simulink model "dqn_C_PQ_HVsMC"  (R2024a)
settings: Solver=FixedStepDiscrete  StartTime=0.0  StopTime=10  FixedStep=Ts_Power  RelTol=1e-3
PreLoadFcn:
  | % HVDCMMCInterconnectionParam
StartFcn:
  | tic
StopFcn:
  | toc
values from neighbouring files (symbols this model uses):
  C_PM = 1.758e-3    (= 0.001758)    [dqnMMCsingle.m]
  Fnom = 50    [dqnMMCsingle.m]
  Ki_Ireg = 6    [dqnMMCsingle.m]
  Ki_Qreg = 1.0    (= 1)    [dqnMMCsingle.m]
  Kp_Ireg = 0.6    [dqnMMCsingle.m]
  Kp_Qreg = 0.5/3    (= 0.166666666667)    [dqnMMCsingle.m]
  Larm = Larm_pu*(Zb_ac/(2*pi*Fnom))    [dqnMMCsingle.m]
  Larm_pu = 0.15    [dqnMMCsingle.m]
  Lff = Larm_pu/2    (= 0.075)    [dqnMMCsingle.m]
  Limits_Ireg = [ 2.0  -2.0]    [dqnMMCsingle.m]
  Limits_Qreg = [ 0.25, -0.25 ]    [dqnMMCsingle.m]
  Limits_VDCreg = [ 2.0  -2.0]    [dqnMMCsingle.m]
  Lxfo = 0.12    [dqnMMCsingle.m]
  N = 1    [dqnMMCsingle.m]
  Nb_PM = 36    [dqnMMCsingle.m]
  Pnom = 1000e6    (= 1000000000)    [dqnMMCsingle.m]
  R_startup = 400    [dqnMMCsingle.m]
  Rarm = Rarm_pu*Zb_ac    [dqnMMCsingle.m]
  Rff = Rarm_pu/2    (= 0.00075)    [dqnMMCsingle.m]
  Rxfo = 0.003    [dqnMMCsingle.m]
  Slope_Qref = 0.5    [dqnMMCsingle.m]
  Slope_Vdc_ref = Vnom_dc/5    (= 128000)    [dqnMMCsingle.m]
  Tfault = 9999    [dqnMMCsingle.m]
  Ts = Ts_Control    (= 4e-05)    [dqnMMCsingle.m]
  Ts_Control = 40e-6    (= 4e-05)    [dqnMMCsingle.m]
  Ts_dqn = 2e-5    (= 2e-05)    [dqnMMCsingle.m]
  Ts_Power = 20e-6    (= 2e-05)    [dqnMMCsingle.m]
  Vnom_dc = 640e3    (= 640000)    [dqnMMCsingle.m]
  Vnom_prim = 400e3    (= 400000)    [dqnMMCsingle.m]
  Vnom_sec = 333e3    (= 333000)    [dqnMMCsingle.m]
undefined symbols (not defined in the file or in its folder): DiscIntNeverNeededParam, Discrete, DQN_Lib, gcbh, HRM, Int_DQNc_Mat, Mult_DQNc_Mat, Pcc, S, sps, sps_rtmsupport, spsMeanValueVariableFrequencyModel, spsPLL3phModel, SY3, Ws
libraries: simulink x18, spsControlledVoltageSourceLib x15, spsVoltageMeasurementLib x9, powerlib_extras x6, spsSecondOrderFilterLib x6, spsCurrentMeasurementLib x6, spsIdealSwitchLib x6, spsMeanLib x4, spsdq0toabcLib x4, spsMeanVariableFrequencyLib x4, spsabctodq0Lib x4, spsThreePhaseSeriesRLCBranchLib x4
(part 4 of 6)

== system dqn_C_PQ_HVsMC/Control _DQn/PLL, Measurements and Transformation1/PLL (3ph)/Model/Variable Frequency Mean value/Model/Correction subsystem ==
  N : Inport
  F : Inport  Port=2
  In : Inport  Port=3
  Gain1 : Gain  Gain=0.5  SaturateOnIntegerOverflow=on  OutDataTypeStr=Inherit: Same as input  ParamDataTypeStr=Inherit: Same as input
  Product2 : Product  Inputs=*/  InputSameDT=on  SaturateOnIntegerOverflow=on  OutDataTypeStr=Inherit: Same as first input
  Product4 : Product  Inputs=**  InputSameDT=on  SaturateOnIntegerOverflow=on  OutDataTypeStr=Inherit: Same as first input
  Product5 : Product  Inputs=**  InputSameDT=on  SaturateOnIntegerOverflow=on  OutDataTypeStr=Inherit: Same as first input
  Sum1 : Sum  Inputs=+-  InputSameDT=on  SaturateOnIntegerOverflow=on  OutDataTypeStr=Inherit: Same as first input
  Sum4 : Sum  InputSameDT=on  SaturateOnIntegerOverflow=on  OutDataTypeStr=Inherit: Same as first input
  Sum5 : Sum  Inputs=+-  InputSameDT=on  SaturateOnIntegerOverflow=on  OutDataTypeStr=Inherit: Same as first input
  Unit Delay : UnitDelay  SampleTime=Ts  HasFrameUpgradeWarning=on
  Out : Outport
  wires:
  Product4/1 -> Out/1
  Sum4/1 -> Product4/2
  Gain1/1 -> Sum4/1
  Product5/1 -> Gain1/1
  Sum1/1 -> Product5/2
  In/1 -> Sum4/2, Unit Delay/1, Sum1/1
  Product2/1 -> Product4/1
  Sum5/1 -> Product5/1, Product2/1
  F/1 -> Sum5/2
  N/1 -> Product2/2, Sum5/1
  Unit Delay/1 -> Sum1/2

== system dqn_C_PQ_HVsMC/Control _DQn/PLL, Measurements and Transformation1/PLL (3ph)2/Model/Variable Frequency Mean value/Model/Correction subsystem ==
  N : Inport
  F : Inport  Port=2
  In : Inport  Port=3
  Gain1 : Gain  Gain=0.5  SaturateOnIntegerOverflow=on  OutDataTypeStr=Inherit: Same as input  ParamDataTypeStr=Inherit: Same as input
  Product2 : Product  Inputs=*/  InputSameDT=on  SaturateOnIntegerOverflow=on  OutDataTypeStr=Inherit: Same as first input
  Product4 : Product  Inputs=**  InputSameDT=on  SaturateOnIntegerOverflow=on  OutDataTypeStr=Inherit: Same as first input
  Product5 : Product  Inputs=**  InputSameDT=on  SaturateOnIntegerOverflow=on  OutDataTypeStr=Inherit: Same as first input
  Sum1 : Sum  Inputs=+-  InputSameDT=on  SaturateOnIntegerOverflow=on  OutDataTypeStr=Inherit: Same as first input
  Sum4 : Sum  InputSameDT=on  SaturateOnIntegerOverflow=on  OutDataTypeStr=Inherit: Same as first input
  Sum5 : Sum  Inputs=+-  InputSameDT=on  SaturateOnIntegerOverflow=on  OutDataTypeStr=Inherit: Same as first input
  Unit Delay : UnitDelay  SampleTime=Ts  HasFrameUpgradeWarning=on
  Out : Outport
  wires:
  Product4/1 -> Out/1
  Sum4/1 -> Product4/2
  Gain1/1 -> Sum4/1
  Product5/1 -> Gain1/1
  Sum1/1 -> Product5/2
  In/1 -> Sum4/2, Unit Delay/1, Sum1/1
  Product2/1 -> Product4/1
  Sum5/1 -> Product5/1, Product2/1
  F/1 -> Sum5/2
  N/1 -> Product2/2, Sum5/1
  Unit Delay/1 -> Sum1/2

== matlab function dqn_C_PQ_HVsMC/DQsym/Subsystem/DQn->ABC11 ==
  settings: updateMethod=DISCRETE
  data: Xdcpnz_c input; tho input; Xabc output; N parameter
%function abc = Mult(Z0,Zdp,Zqp,Zdn,Zqn,Zdz,Zqz,th, N)
function Xabc = dqn2abc(Xdcpnz_c,tho,N)

    persistent Sas;
    persistent Ssa;

    if(isempty(Sas)) 
        a = -0.5+0.866i;
        a2 = -0.5-0.866i;
        Sas = [1,a,a2;1,a2,a;1,1,1]/3;
        Ssa = eye(3)/(Sas);
    end

    Xabc = zeros(3,1);

    for i = 1 : N+1
    
    
        if(i>1)
            h = i-1;
    
            th = h*tho;
        
            mag_p = abs(Xdcpnz_c(1,i));
            ang_p = angle(Xdcpnz_c(1,i));
            mag_n = abs(Xdcpnz_c(2,i));
            ang_n = angle(Xdcpnz_c(2,i));
            mag_z = abs(Xdcpnz_c(3,i));
            ang_z = angle(Xdcpnz_c(3,i));
            
            abc3p = mag_p*[sin(th+ang_p) ; sin(th+ang_p-2*pi/3) ; sin(th+ang_p+2*pi/3) ];
            abc3n = mag_n*[sin(th+ang_n) ; sin(th+ang_n+2*pi/3) ; sin(th+ang_n-2*pi/3) ];
            abc3z = mag_z*[sin(th+ang_z) ; sin(th+ang_z)        ; sin(th+ang_z)  ];
        
            Xabc = Xabc + abc3p+abc3n+abc3z;
        else
            Xabc = Xabc + real(Ssa*(Xdcpnz_c(:,1)));
        
        end
    
        
    end

end

== matlab function dqn_C_PQ_HVsMC/DQsym/Subsystem/DQn->ABC12 ==
  settings: updateMethod=DISCRETE
  data: Xdcpnz_c input; tho input; Xabc output; N parameter
%function abc = Mult(Z0,Zdp,Zqp,Zdn,Zqn,Zdz,Zqz,th, N)
function Xabc = dqn2abc(Xdcpnz_c,tho,N)

    persistent Sas;
    persistent Ssa;

    if(isempty(Sas)) 
        a = -0.5+0.866i;
        a2 = -0.5-0.866i;
        Sas = [1,a,a2;1,a2,a;1,1,1]/3;
        Ssa = eye(3)/(Sas);
    end

    Xabc = zeros(3,1);

    for i = 1 : N+1
    
    
        if(i>1)
            h = i-1;
    
            th = h*tho;
        
            mag_p = abs(Xdcpnz_c(1,i));
            ang_p = angle(Xdcpnz_c(1,i));
            mag_n = abs(Xdcpnz_c(2,i));
            ang_n = angle(Xdcpnz_c(2,i));
            mag_z = abs(Xdcpnz_c(3,i));
            ang_z = angle(Xdcpnz_c(3,i));
            
            abc3p = mag_p*[sin(th+ang_p) ; sin(th+ang_p-2*pi/3) ; sin(th+ang_p+2*pi/3) ];
            abc3n = mag_n*[sin(th+ang_n) ; sin(th+ang_n+2*pi/3) ; sin(th+ang_n-2*pi/3) ];
            abc3z = mag_z*[sin(th+ang_z) ; sin(th+ang_z)        ; sin(th+ang_z)  ];
        
            Xabc = Xabc + abc3p+abc3n+abc3z;
        else
            Xabc = Xabc + real(Ssa*(Xdcpnz_c(:,1)));
        
        end
    
        
    end

end

== matlab function dqn_C_PQ_HVsMC/DQsym/Subsystem/DQn->ABC13 ==
  settings: updateMethod=DISCRETE
  data: Xdcpnz_c input; tho input; Xabc output; N parameter
%function abc = Mult(Z0,Zdp,Zqp,Zdn,Zqn,Zdz,Zqz,th, N)
function Xabc = dqn2abc(Xdcpnz_c,tho,N)

    persistent Sas;
    persistent Ssa;

    if(isempty(Sas)) 
        a = -0.5+0.866i;
        a2 = -0.5-0.866i;
        Sas = [1,a,a2;1,a2,a;1,1,1]/3;
        Ssa = eye(3)/(Sas);
    end

    Xabc = zeros(3,1);

    for i = 1 : N+1
    
    
        if(i>1)
            h = i-1;
    
            th = h*tho;
        
            mag_p = abs(Xdcpnz_c(1,i));
            ang_p = angle(Xdcpnz_c(1,i));
            mag_n = abs(Xdcpnz_c(2,i));
            ang_n = angle(Xdcpnz_c(2,i));
            mag_z = abs(Xdcpnz_c(3,i));
            ang_z = angle(Xdcpnz_c(3,i));
            
            abc3p = mag_p*[sin(th+ang_p) ; sin(th+ang_p-2*pi/3) ; sin(th+ang_p+2*pi/3) ];
            abc3n = mag_n*[sin(th+ang_n) ; sin(th+ang_n+2*pi/3) ; sin(th+ang_n-2*pi/3) ];
            abc3z = mag_z*[sin(th+ang_z) ; sin(th+ang_z)        ; sin(th+ang_z)  ];
        
            Xabc = Xabc + abc3p+abc3n+abc3z;
        else
            Xabc = Xabc + real(Ssa*(Xdcpnz_c(:,1)));
        
        end
    
        
    end

end

== matlab function dqn_C_PQ_HVsMC/DQsym/Subsystem/DQn->ABC14 ==
  settings: updateMethod=DISCRETE
  data: Xdcpnz_c input; tho input; Xabc output; N parameter
%function abc = Mult(Z0,Zdp,Zqp,Zdn,Zqn,Zdz,Zqz,th, N)
function Xabc = dqn2abc(Xdcpnz_c,tho,N)

    persistent Sas;
    persistent Ssa;

    if(isempty(Sas)) 
        a = -0.5+0.866i;
        a2 = -0.5-0.866i;
        Sas = [1,a,a2;1,a2,a;1,1,1]/3;
        Ssa = eye(3)/(Sas);
    end

    Xabc = zeros(3,1);

    for i = 1 : N+1
    
    
        if(i>1)
            h = i-1;
    
            th = h*tho;
        
            mag_p = abs(Xdcpnz_c(1,i));
            ang_p = angle(Xdcpnz_c(1,i));
            mag_n = abs(Xdcpnz_c(2,i));
            ang_n = angle(Xdcpnz_c(2,i));
            mag_z = abs(Xdcpnz_c(3,i));
            ang_z = angle(Xdcpnz_c(3,i));
            
            abc3p = mag_p*[sin(th+ang_p) ; sin(th+ang_p-2*pi/3) ; sin(th+ang_p+2*pi/3) ];
            abc3n = mag_n*[sin(th+ang_n) ; sin(th+ang_n+2*pi/3) ; sin(th+ang_n-2*pi/3) ];
            abc3z = mag_z*[sin(th+ang_z) ; sin(th+ang_z)        ; sin(th+ang_z)  ];
        
            Xabc = Xabc + abc3p+abc3n+abc3z;
        else
            Xabc = Xabc + real(Ssa*(Xdcpnz_c(:,1)));
        
        end
    
        
    end

end

== matlab function dqn_C_PQ_HVsMC/DQsym/Subsystem/DQn->ABC15 ==
  settings: updateMethod=DISCRETE
  data: Xdcpnz_c input; tho input; Xabc output; N parameter
%function abc = Mult(Z0,Zdp,Zqp,Zdn,Zqn,Zdz,Zqz,th, N)
function Xabc = dqn2abc(Xdcpnz_c,tho,N)

    persistent Sas;
    persistent Ssa;

    if(isempty(Sas)) 
        a = -0.5+0.866i;
        a2 = -0.5-0.866i;
        Sas = [1,a,a2;1,a2,a;1,1,1]/3;
        Ssa = eye(3)/(Sas);
    end

    Xabc = zeros(3,1);

    for i = 1 : N+1
    
    
        if(i>1)
            h = i-1;
    
            th = h*tho;
        
            mag_p = abs(Xdcpnz_c(1,i));
            ang_p = angle(Xdcpnz_c(1,i));
            mag_n = abs(Xdcpnz_c(2,i));
            ang_n = angle(Xdcpnz_c(2,i));
            mag_z = abs(Xdcpnz_c(3,i));
            ang_z = angle(Xdcpnz_c(3,i));
            
            abc3p = mag_p*[sin(th+ang_p) ; sin(th+ang_p-2*pi/3) ; sin(th+ang_p+2*pi/3) ];
            abc3n = mag_n*[sin(th+ang_n) ; sin(th+ang_n+2*pi/3) ; sin(th+ang_n-2*pi/3) ];
            abc3z = mag_z*[sin(th+ang_z) ; sin(th+ang_z)        ; sin(th+ang_z)  ];
        
            Xabc = Xabc + abc3p+abc3n+abc3z;
        else
            Xabc = Xabc + real(Ssa*(Xdcpnz_c(:,1)));
        
        end
    
        
    end

end

== matlab function dqn_C_PQ_HVsMC/DQsym/Subsystem/DQn->ABC16 ==
  settings: updateMethod=DISCRETE
  data: Xdcpnz_c input; tho input; Xabc output; N parameter
%function abc = Mult(Z0,Zdp,Zqp,Zdn,Zqn,Zdz,Zqz,th, N)
function Xabc = dqn2abc(Xdcpnz_c,tho,N)

    persistent Sas;
    persistent Ssa;

    if(isempty(Sas)) 
        a = -0.5+0.866i;
        a2 = -0.5-0.866i;
        Sas = [1,a,a2;1,a2,a;1,1,1]/3;
        Ssa = eye(3)/(Sas);
    end

    Xabc = zeros(3,1);

    for i = 1 : N+1
    
    
        if(i>1)
            h = i-1;
    
            th = h*tho;
        
            mag_p = abs(Xdcpnz_c(1,i));
            ang_p = angle(Xdcpnz_c(1,i));
            mag_n = abs(Xdcpnz_c(2,i));
            ang_n = angle(Xdcpnz_c(2,i));
            mag_z = abs(Xdcpnz_c(3,i));
            ang_z = angle(Xdcpnz_c(3,i));
            
            abc3p = mag_p*[sin(th+ang_p) ; sin(th+ang_p-2*pi/3) ; sin(th+ang_p+2*pi/3) ];
            abc3n = mag_n*[sin(th+ang_n) ; sin(th+ang_n+2*pi/3) ; sin(th+ang_n-2*pi/3) ];
            abc3z = mag_z*[sin(th+ang_z) ; sin(th+ang_z)        ; sin(th+ang_z)  ];
        
            Xabc = Xabc + abc3p+abc3n+abc3z;
        else
            Xabc = Xabc + real(Ssa*(Xdcpnz_c(:,1)));
        
        end
    
        
    end

end

== matlab function dqn_C_PQ_HVsMC/DQsym/Subsystem/DQn->ABC17 ==
  settings: updateMethod=DISCRETE
  data: Xdcpnz_c input; tho input; Xabc output; N parameter
%function abc = Mult(Z0,Zdp,Zqp,Zdn,Zqn,Zdz,Zqz,th, N)
function Xabc = dqn2abc(Xdcpnz_c,tho,N)

    persistent Sas;
    persistent Ssa;

    if(isempty(Sas)) 
        a = -0.5+0.866i;
        a2 = -0.5-0.866i;
        Sas = [1,a,a2;1,a2,a;1,1,1]/3;
        Ssa = eye(3)/(Sas);
    end

    Xabc = zeros(3,1);

    for i = 1 : N+1
    
    
        if(i>1)
            h = i-1;
    
            th = h*tho;
        
            mag_p = abs(Xdcpnz_c(1,i));
            ang_p = angle(Xdcpnz_c(1,i));
            mag_n = abs(Xdcpnz_c(2,i));
            ang_n = angle(Xdcpnz_c(2,i));
            mag_z = abs(Xdcpnz_c(3,i));
            ang_z = angle(Xdcpnz_c(3,i));
            
            abc3p = mag_p*[sin(th+ang_p) ; sin(th+ang_p-2*pi/3) ; sin(th+ang_p+2*pi/3) ];
            abc3n = mag_n*[sin(th+ang_n) ; sin(th+ang_n+2*pi/3) ; sin(th+ang_n-2*pi/3) ];
            abc3z = mag_z*[sin(th+ang_z) ; sin(th+ang_z)        ; sin(th+ang_z)  ];
        
            Xabc = Xabc + abc3p+abc3n+abc3z;
        else
            Xabc = Xabc + real(Ssa*(Xdcpnz_c(:,1)));
        
        end
    
        
    end

end

== matlab function dqn_C_PQ_HVsMC/DQsym/Subsystem/DQn->ABC8 ==
  settings: updateMethod=DISCRETE
  data: Xdcpnz_c input; tho input; Xabc output; N parameter
%function abc = Mult(Z0,Zdp,Zqp,Zdn,Zqn,Zdz,Zqz,th, N)
function Xabc = dqn2abc(Xdcpnz_c,tho,N)

    persistent Sas;
    persistent Ssa;

    if(isempty(Sas)) 
        a = -0.5+0.866i;
        a2 = -0.5-0.866i;
        Sas = [1,a,a2;1,a2,a;1,1,1]/3;
        Ssa = eye(3)/(Sas);
    end

    Xabc = zeros(3,1);

    for i = 1 : N+1
    
    
        if(i>1)
            h = i-1;
    
            th = h*tho;
        
            mag_p = abs(Xdcpnz_c(1,i));
            ang_p = angle(Xdcpnz_c(1,i));
            mag_n = abs(Xdcpnz_c(2,i));
            ang_n = angle(Xdcpnz_c(2,i));
            mag_z = abs(Xdcpnz_c(3,i));
            ang_z = angle(Xdcpnz_c(3,i));
            
            abc3p = mag_p*[sin(th+ang_p) ; sin(th+ang_p-2*pi/3) ; sin(th+ang_p+2*pi/3) ];
            abc3n = mag_n*[sin(th+ang_n) ; sin(th+ang_n+2*pi/3) ; sin(th+ang_n-2*pi/3) ];
            abc3z = mag_z*[sin(th+ang_z) ; sin(th+ang_z)        ; sin(th+ang_z)  ];
        
            Xabc = Xabc + abc3p+abc3n+abc3z;
        else
            Xabc = Xabc + real(Ssa*(Xdcpnz_c(:,1)));
        
        end
    
        
    end

end

== matlab function dqn_C_PQ_HVsMC/DQsym/DQsym_SS ==
  data: Ad parameter; Bd parameter; Cd parameter; Dd parameter; swOnRes parameter; swOffRes parameter; swType parameter; brkVec input; y output [1..100]; u input; xo input
function y  = nFdss2(Ad, Bd, Cd, Dd, swOnRes, swOffRes, swType, brkVec, u,xo)

% INIT


persistent Ads;
persistent Bds;
persistent Cds;
persistent Dds;
persistent x;
persistent x_old;
persistent swVec;
persistent swVecOld;
persistent nSwitches;
persistent nStates;
persistent nOutputs;
persistent nInputs;
persistent yswitch;
persistent xkm12;   % First half-step state at t - Ts/2
persistent xkp12;   % Second half-step state at t + Ts/2
persistent xCorrected; % Corrected state at time t


x = complex(zeros(size(Ad,1),size(u,2)));
y = complex(zeros(size(Cd,1),size(u,2)));


% Adc= Ad; Bdc = Bd ; Cdc = Cd; Ddc = Dd;

[Adc, Bdc, Cdc, Ddc] = convertToPhasor(Ad, Bd, Cd, Dd);
% Initialization (First Call)

if isempty(x_old)

    if (swType ~= 0)
    
        nStates = size(Ad, 1);
        nInputs = size(Bd, 2);
        nOutputs = size(Cd, 1);
        nSwitches = sum(swType == 1);

        x_old = complex([xo,zeros(size(xo,1),size(u,2)-1)]);
        xCorrected = x_old;

        swVec = brkVec;
        swVecOld = swVec;

        yswitch = complex(zeros(nSwitches));


        xkp12 = complex(zeros(nStates, 1));
        xkm12 = complex(zeros(nStates, 1));

         % First Half-step Correction: xkm12 at t - Ts/2 % Before Updating Matrices

            % Calculate using old state (x_old) and unmodified matrices (Ads, Bds)
            for j = 1:nStates
                for i = 1:nStates
                    if i == j
                        xkm12(i) = xkm12(i) + (Adc(i, j) + 1) * 0.5 * x_old(j);
                    else
                        xkm12(i) = xkm12(i) + Adc(i, j) * 0.5 * x_old(j);
                    end
                end
            end

            % Matrix B Contribution for First Half-step
            for j = 1:nInputs
                for i = 1:nStates
                    xkm12(i) = xkm12(i) + Bdc(i, j) * 0.5 * u(j);
                end
            end


    
        % Detect switch changes
        SwitchChange = (swVecOld ~= swVec);
        idxSwChng = find(SwitchChange == 1); % Indices of changed switches
        nbSwChng = sum(SwitchChange == 1);   % Number of switches that changed

        % Update switching conductance
        for s = 1:nSwitches
            if swVec(s) == 1
                yswitch(s) = complex(1 / swOnRes(s));
            else
                yswitch(s) = complex(1 / swOffRes(s));
            end
        end

        % Initialize DxCol and BDcol (for matrix updates)
        DxCol = complex(zeros(nOutputs, 1));
        BDcol = complex(zeros(nStates, 1));

        % Process each switch change
        for k = 1:nbSwChng
            nSw = idxSwChng(k);  % Get switch index
            kSw = SwitchChange(nSw);  % Get new switch state

            % Compute DxCol update for D matrix
            tmp = Ddc(nSw, nSw) * yswitch(nSw);
            temp = complex(1 / (1 - tmp * kSw));
            temp2 = yswitch(nSw) * temp * kSw;

            for i = 1:nOutputs
                DxCol(i) = Ddc(i, nSw) * temp2;
            end
            DxCol(nSw) = temp;

            % Compute BDcol update for B matrix
            temp2 = yswitch(nSw) * kSw;
            for i = 1:nStates
                BDcol(i) = Bdc(i, nSw) * temp2;
            end

            % Copy row nSw of Cd and zero it out
            tmp1 = Cdc(nSw, :);
            Cdc(nSw, :) = complex(0);

            % Copy row nSw of Dd and zero it out
            tmp2 = Ddc(nSw, :);
            Ddc(nSw, :) = complex(0);

            % Update C and D matrices
            for i = 1:nOutputs
                for j = 1:nStates
                    Cdc(i, j) = Cdc(i, j) + DxCol(i) * tmp1(j);
                end
                for j = 1:nInputs
                    Ddc(i, j) = Ddc(i, j) + DxCol(i) * tmp2(j);
                end
            end

            % Update A and B matrices
            for i = 1:nStates
                for j = 1:nStates
                    Adc(i, j) = Adc(i, j) + BDcol(i) * Cdc(nSw, j);
                end
                for j = 1:nInputs
                    Bdc(i, j) = Bdc(i, j) + BDcol(i) * Ddc(nSw, j);
                end
            end
        end


        % Store updated matrices
        Ads = Adc;
        Bds = Bdc;
        Cds = Cdc;
        Dds = Ddc;

           % SECOND HALF-STEP CORRECTION % After Updating Matrices


            for j = 1:nStates
                for i = 1:nStates
                    if i == j
                        xkp12(i) = xkp12(i) + (Ads(i, j) + 1) * 0.5 * x_old(j);
                    else
                        xkp12(i) = xkp12(i) + Ads(i, j) * 0.5 * x_old(j);
                    end
                end
            end

            % Matrix B Contribution for Second Half-step
            for j = 1:nInputs
                for i = 1:nStates
                    xkp12(i) = xkp12(i) + Bds(i, j) * 0.5 * u(j);
                end
            end


    % Store old switch vector for next iteration
        swVecOld = swVec;

        x_old(:,1) = (xkp12 + xkm12) * 0.5;

     else
        nStates = size(Ad, 1);
        nInputs = size(Bd, 2);
        nOutputs = size(Cd, 1);
        nSwitches = sum(swType == 1);

        x_old = complex([xo,zeros(size(xo,1),size(u,2)-1)]);
        xCorrected = x_old;

        swVec = brkVec;
        swVecOld = swVec;

        Ads = Adc;
        Bds = Bdc;
        Cds = Cdc;
        Dds = Ddc;
    end
end

% Update switch vector
if (swType ~= 0)
    swVec = brkVec;
end


% DETECT SWITCH CHANGES AND UPDATE MATRICES

if (any(swType ~= 0) && any(swVecOld ~= swVec))

        nStates = size(Ad, 1);
        nInputs = size(Bd, 2);
        nOutputs = size(Cd, 1);
        nSwitches = sum(swType == 1);
        
        yswitch = complex(zeros(nSwitches));

        xkp12 = complex(zeros(nStates, 1));
        xkm12 = complex(zeros(nStates, 1));

        % First Half-step Correction: xkm12 at t - Ts/2 % Before Updating Matrices

            % Calculate using old state (x_old) and unmodified matrices (Ads, Bds)
            for j = 1:nStates
                for i = 1:nStates
                    if i == j
                        xkm12(i) = xkm12(i) + (Ads(i, j) + 1) * 0.5 * x_old(j);
                    else
                        xkm12(i) = xkm12(i) + Ads(i, j) * 0.5 * x_old(j);
                    end
                end
            end

            % Matrix B Contribution for First Half-step
            for j = 1:nInputs
                for i = 1:nStates
                    xkm12(i) = xkm12(i) + Bds(i, j) * 0.5 * u(j);
                end
            end



       % Detect switch changes
        SwitchChange = (swVecOld ~= swVec);
        idxSwChng = find(SwitchChange == 1); % Indices of changed switches
        nbSwChng = sum(SwitchChange == 1);   % Number of switches that changed

        % Update switching conductance
        for s = 1:nSwitches
            if swVec(s) == 1
                yswitch(s) = complex(1 / swOnRes(s));
            else
                yswitch(s) = complex(1 / swOffRes(s));
            end
        end

        % Initialize DxCol and BDcol (for matrix updates)
        DxCol = complex(zeros(nOutputs, 1));
        BDcol = complex(zeros(nStates, 1));

        % Process each switch change
        for k = 1:nbSwChng
            nSw = idxSwChng(k);  % Get switch index
            kSw = SwitchChange(nSw);  % Get new switch state

            % Compute DxCol update for D matrix
            tmp = Dds(nSw, nSw) * yswitch(nSw);
            temp = complex(1 / (1 - tmp * kSw));
            temp2 = yswitch(nSw) * temp * kSw;

            for i = 1:nOutputs
                DxCol(i) = Dds(i, nSw) * temp2;
            end
            DxCol(nSw) = temp;

            % Compute BDcol update for B matrix
            temp2 = yswitch(nSw) * kSw;
            for i = 1:nStates
                BDcol(i) = Bds(i, nSw) * temp2;
            end

            % Copy row nSw of Cd and zero it out
            tmp1 = Cds(nSw, :);
            Cds(nSw, :) = complex(0);

            % Copy row nSw of Dd and zero it out
            tmp2 = Dds(nSw, :);
            Dds(nSw, :) = complex(0);

            % Update C and D matrices
            for i = 1:nOutputs
                for j = 1:nStates
                    Cds(i, j) = Cds(i, j) + DxCol(i) * tmp1(j);
                end
                for j = 1:nInputs
                    Dds(i, j) = Dds(i, j) + DxCol(i) * tmp2(j);
                end
            end

            % Update A and B matrices
            for i = 1:nStates
                for j = 1:nStates
                    Ads(i, j) = Ads(i, j) + BDcol(i) * Cds(nSw, j);
                end
                for j = 1:nInputs
                    Bds(i, j) = Bds(i, j) + BDcol(i) * Dds(nSw, j);
                end
            end
        end


        % Store updated matrices
        % Ads;
        % Bds;
        % Cds;
        % Dds;

            
        % SECOND HALF-STEP CORRECTION % After Updating Matrices


            for j = 1:nStates
                for i = 1:nStates
                    if i == j
                        xkp12(i) = xkp12(i) + (Ads(i, j) + 1) * 0.5 * x_old(j);
                    else
                        xkp12(i) = xkp12(i) + Ads(i, j) * 0.5 * x_old(j);
                    end
                end
            end

            % Matrix B Contribution for Second Half-step
            for j = 1:nInputs
                for i = 1:nStates
                    xkp12(i) = xkp12(i) + Bds(i, j) * 0.5 * u(j);
                end
            end

    % Store old switch vector for next iteration
        swVecOld = swVec;

         x_old(:,1) = (xkp12 + xkm12) * 0.5;

end 
   
       % Ao=Ads;
       % Bo=Bds;
       % Co=Cds;
       % Do=Dds;


% STATE AND OUTPUT CALCULATION
x = Ads * x_old + Bds * u;

 x2= x *  diag(exp(-[0:(size(u,2)-1)].*2*pi*50*2e-5*1i));

x_old= x2;

% xout=xCorrected;

y = Cds * x2 + Dds * u;

end


function [Adc1, Bdc1, Cdc1, Ddc1] = convertToPhasor(A, B, C, D)

    dt= 2e-5;

    % Step 1: Discretize the matrices
    I = eye(size(A, 1));
    Ad1 = inv(I - (dt * A / 2)) * (I + (dt * A / 2));
    Bd1 = inv(I - (dt * A / 2)) * B * sqrt(dt);
    Cd1 = sqrt(dt) * C * inv(I - (dt * A / 2));
    Dd1 = D + C * inv(I - (dt * A / 2)) * (B * dt / 2);

    % 
    % Ad2= Ad1; Bd2 = Bd1; Cd2 = Cd1 ; Dd2= Dd1; 
    Ad2= A; Bd2 = B; Cd2 = C ; Dd2= D; %%temp for testing without TBE dis

    %Convert to DQN
    a = -0.5 + 0.866i;
    a2 = -0.5 - 0.866i;
    Sas = [1, a, a2; 1, a2, a; 1, 1, 1] / 3;

    % Perform the phasor transformation for each matrix
    Adc1 = transformMatrix(Ad2, Sas);
    Bdc1 = transformMatrix(Bd2, Sas);
    Cdc1 = transformMatrix(Cd2, Sas);
    Ddc1 = transformMatrix(Dd2, Sas);

end

function Mdc = transformMatrix(Md1, Sas)
    [rows, cols] = size(Md1);
    rows = rows / 3;
    cols = cols / 3;
    Mdc = complex(zeros(3 * rows, 3 * cols));
    for i = 1:rows
        for j = 1:cols
            Mdc((1:3) + (i - 1) * 3, (1:3) + (j - 1) * 3) = ...
                Sas * Md1((1:3) + (i - 1) * 3, (1:3) + (j - 1) * 3) / Sas;
        end
    end
end

== matlab function dqn_C_PQ_HVsMC/DQsym/Int_DQNc_Mat1 ==
  settings: updateMethod=DISCRETE
  data: Xpnz input; N parameter; dt parameter; w parameter; InitInt parameter; Zpnz output; R parameter; iL parameter; swFeed parameter
function Zpnz    = Int_DQN_Mat(Xpnz, N, dt, w, InitInt, R, iL, swFeed)


    nrSig = size(Xpnz,1)/3;
    Zpnz = complex(zeros(nrSig*3,N+1));

    persistent Zpnz_old;
    persistent Xpnz_old;
    persistent Krl1;
    persistent Krl2;
    persistent dt2;
        
    if(isempty(Zpnz_old)) 
    


        
        % if(~isempty(InitInt))
        % Zpnz_old(:,1) = Sas * InitInt;
        % end


        Zpnz_old = complex(zeros(nrSig*3,N+1));
        Xpnz_old = complex(zeros(nrSig*3,N+1));
        dt2 = dt/2;

        if(swFeed)
            mrows = size(R,1)/3; %signal size
            mcols = size(R,2)/3; %signal size

            szMatR = size(R,1);
            szMatiL = size(iL,1);

            if(szMatiL ~= szMatR || size(R,1) ~= size(R,2) || size(iL,1) ~= size(iL,2))
                error('[Int_DQN_Mat/swFeedback] check matrix sizes!');
            end
    
            Rpnz = complex(zeros(3*mrows,3*mcols));
            iLpnz = complex(zeros(3*mrows,3*mcols));

            a = -0.5+0.866i;
            a2 = -0.5-0.866i;
            Sas = [1,a,a2;1,a2,a;1,1,1]/3;
    
            for i = 1 : mrows
                for j = 1 : mcols
                     Rpnz((1:3) + (i-1)*3,(1:3) + (j-1)*3) = Sas*R((1:3) + (i-1)*3,(1:3) + (j-1)*3)/Sas;
                    iLpnz((1:3) + (i-1)*3,(1:3) + (j-1)*3) = Sas*iL((1:3) + (i-1)*3,(1:3) + (j-1)*3)/Sas;
                end
            end

            Rpnz  = diag(diag(real(Rpnz)));
            iLpnz = diag(diag(real(iLpnz)));

            Krl1 = (iLpnz/(eye(szMatR)+dt2*Rpnz*iLpnz));
            Krl2 = (eye(szMatR)-dt2*Rpnz*iLpnz)/(eye(szMatR)+dt2*Rpnz*iLpnz);
        else
            Krl1 = 1;
            Krl2 = 1;
        end
            
    end

    if(swFeed)
        Zpnz(:,1) = Krl1*dt2*(Xpnz(:,1)+Xpnz_old(:,1))+Krl2*Zpnz_old(:,1);
    else
        Zpnz(:,1) = dt2*(Xpnz(:,1)+Xpnz_old(:,1))+Zpnz_old(:,1);
    end

    Xpnz_old(:,1) = Xpnz(:,1);
    Zpnz_old(:,1) = Zpnz(:,1);

    for i = 1 : N
        if(N>0)
            wn =  i * w; 
            wndt2 = wn*dt2;

            A = 2*dt2/(1+wndt2^2);
            B = (1-wndt2^2)/(1+wndt2^2);

            if(swFeed)

                Zpnz(:,i+1) =      Krl1*A*(real(Xpnz(:,i+1))+wndt2*imag(Xpnz(:,i+1)))+Krl2*(B*real(Zpnz_old(:,i+1))+A*wn*imag(Zpnz_old(:,i+1))) ...
                             + 1i*(Krl1*A*(imag(Xpnz(:,i+1))-wndt2*real(Xpnz(:,i+1)))+Krl2*(B*imag(Zpnz_old(:,i+1))-A*wn*real(Zpnz_old(:,i+1))));
            else
                Zpnz(:,i+1) =      A*(real(Xpnz(:,i+1))+wndt2*imag(Xpnz(:,i+1)))+(B*real(Zpnz_old(:,i+1))+A*wn*imag(Zpnz_old(:,i+1))) ...
                             + 1i*(A*(imag(Xpnz(:,i+1))-wndt2*real(Xpnz(:,i+1)))+(B*imag(Zpnz_old(:,i+1))-A*wn*real(Zpnz_old(:,i+1))));
            end

            Zpnz_old(:,i+1) = Zpnz(:,i+1);

        end
    end


end

== matlab function dqn_C_PQ_HVsMC/DQsym/Int_DQNc_Mat2 ==
  settings: updateMethod=DISCRETE
  data: Xpnz input; N parameter; dt parameter; w parameter; InitInt parameter; Zpnz output; R parameter; iL parameter; swFeed parameter
function Zpnz    = Int_DQN_Mat(Xpnz, N, dt, w, InitInt, R, iL, swFeed)


    nrSig = size(Xpnz,1)/3;
    Zpnz = complex(zeros(nrSig*3,N+1));

    persistent Zpnz_old;
    persistent Xpnz_old;
    persistent Krl1;
    persistent Krl2;
    persistent dt2;
        
    if(isempty(Zpnz_old)) 
    


        
        % if(~isempty(InitInt))
        % Zpnz_old(:,1) = Sas * InitInt;
        % end


        Zpnz_old = complex(zeros(nrSig*3,N+1));
        Xpnz_old = complex(zeros(nrSig*3,N+1));
        dt2 = dt/2;

        if(swFeed)
            mrows = size(R,1)/3; %signal size
            mcols = size(R,2)/3; %signal size

            szMatR = size(R,1);
            szMatiL = size(iL,1);

            if(szMatiL ~= szMatR || size(R,1) ~= size(R,2) || size(iL,1) ~= size(iL,2))
                error('[Int_DQN_Mat/swFeedback] check matrix sizes!');
            end
    
            Rpnz = complex(zeros(3*mrows,3*mcols));
            iLpnz = complex(zeros(3*mrows,3*mcols));

            a = -0.5+0.866i;
            a2 = -0.5-0.866i;
            Sas = [1,a,a2;1,a2,a;1,1,1]/3;
    
            for i = 1 : mrows
                for j = 1 : mcols
                     Rpnz((1:3) + (i-1)*3,(1:3) + (j-1)*3) = Sas*R((1:3) + (i-1)*3,(1:3) + (j-1)*3)/Sas;
                    iLpnz((1:3) + (i-1)*3,(1:3) + (j-1)*3) = Sas*iL((1:3) + (i-1)*3,(1:3) + (j-1)*3)/Sas;
                end
            end

            Rpnz  = diag(diag(real(Rpnz)));
            iLpnz = diag(diag(real(iLpnz)));

            Krl1 = (iLpnz/(eye(szMatR)+dt2*Rpnz*iLpnz));
            Krl2 = (eye(szMatR)-dt2*Rpnz*iLpnz)/(eye(szMatR)+dt2*Rpnz*iLpnz);
        else
            Krl1 = 1;
            Krl2 = 1;
        end
            
    end

    if(swFeed)
        Zpnz(:,1) = Krl1*dt2*(Xpnz(:,1)+Xpnz_old(:,1))+Krl2*Zpnz_old(:,1);
    else
        Zpnz(:,1) = dt2*(Xpnz(:,1)+Xpnz_old(:,1))+Zpnz_old(:,1);
    end

    Xpnz_old(:,1) = Xpnz(:,1);
    Zpnz_old(:,1) = Zpnz(:,1);

    for i = 1 : N
        if(N>0)
            wn =  i * w; 
            wndt2 = wn*dt2;

            A = 2*dt2/(1+wndt2^2);
            B = (1-wndt2^2)/(1+wndt2^2);

            if(swFeed)

                Zpnz(:,i+1) =      Krl1*A*(real(Xpnz(:,i+1))+wndt2*imag(Xpnz(:,i+1)))+Krl2*(B*real(Zpnz_old(:,i+1))+A*wn*imag(Zpnz_old(:,i+1))) ...
                             + 1i*(Krl1*A*(imag(Xpnz(:,i+1))-wndt2*real(Xpnz(:,i+1)))+Krl2*(B*imag(Zpnz_old(:,i+1))-A*wn*real(Zpnz_old(:,i+1))));
            else
                Zpnz(:,i+1) =      A*(real(Xpnz(:,i+1))+wndt2*imag(Xpnz(:,i+1)))+(B*real(Zpnz_old(:,i+1))+A*wn*imag(Zpnz_old(:,i+1))) ...
                             + 1i*(A*(imag(Xpnz(:,i+1))-wndt2*real(Xpnz(:,i+1)))+(B*imag(Zpnz_old(:,i+1))-A*wn*real(Zpnz_old(:,i+1))));
            end

            Zpnz_old(:,i+1) = Zpnz(:,i+1);

        end
    end


end
